simulink model "rover_bot_obstacles_R2018a"  (R2018a)
settings: Solver=ode23t  StartTime=0.0  StopTime=60  RelTol=1e-3
model workspace (MATLAB code in the model file):
  | a=3;
  | SplinePoints=[-a, -a
  |     -0.904*a, -1.019*a,
  |     -0.8*a, -a
  |     0, -0.9*a
  |     a, -a
  |     0.9*a, 0
  |     a, a
  |     0, 0.9*a
  |     -a, a
  |     -0.9*a, 0
  |     -a, -0.8*a
  |     -1.019*a, -0.904*a];
values from neighbouring files (symbols this model uses):
  m = size(mapxy,1)    [distance2curveSimplified.m]
undefined symbols (not defined in the file or in its folder): distance2curveKH, X, Y, Z
libraries: sm_lib x42, nesl_utility x16
(part 3 of 3)

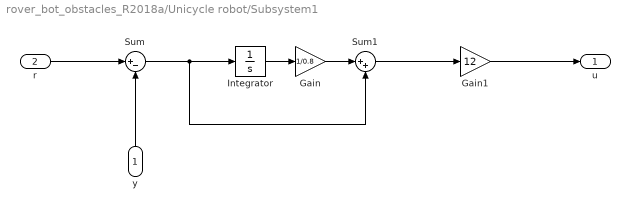
== system rover_bot_obstacles_R2018a/Unicycle robot/Subsystem1 ==
  y : Inport
  r : Inport  Port=2
  Gain : Gain  Gain=1/0.8
  Gain1 : Gain  Gain=12
  Integrator : Integrator
  Sum : Sum  Inputs=|+-
  Sum1 : Sum  Inputs=|++
  u : Outport
  wires:
  Integrator/1 -> Gain/1
  Sum/1 -> Sum1/2, Integrator/1
  r/1 -> Sum/1
  y/1 -> Sum/2
  Gain/1 -> Sum1/1
  Sum1/1 -> Gain1/1
  Gain1/1 -> u/1
